simulink model "simple_dsp_module"  (R2018a)
settings: Solver=VariableStepAuto  StartTime=0.0  StopTime=100e-6  RelTol=1e-3
values from neighbouring files (symbols this model uses):
  BASELINE = 0    [dsp_blr.mat]
libraries: xbsIndex_r4 x84, xrbsSSR_Library x15, simulink x3, dspsigattribs x1, hdlsllib x1
(part 2 of 2)

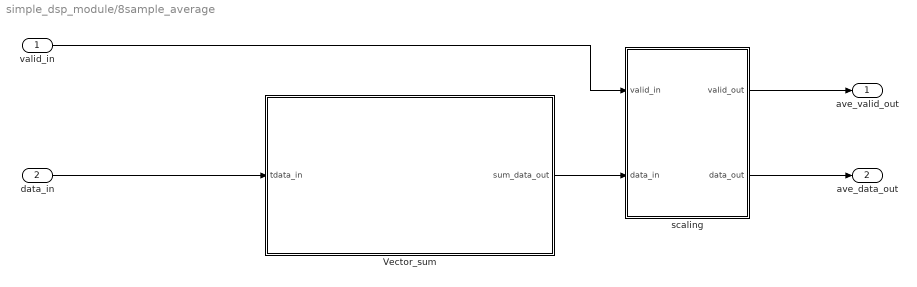
== system simple_dsp_module/8sample_average  ==
  valid_in : Inport
  data_in : Inport  Port=2
  Vector_sum : Subsystem
  scaling : Subsystem
  ave_valid_out : Outport
  ave_data_out : Outport  Port=2
  wires:
  valid_in/1 -> scaling/1(valid_in)
  Vector_sum/1(sum_data_out) -> scaling/2(data_in)
  scaling/2(data_out) -> ave_data_out/1
  data_in/1 -> Vector_sum/1(tdata_in)
  scaling/1(valid_out) -> ave_valid_out/1

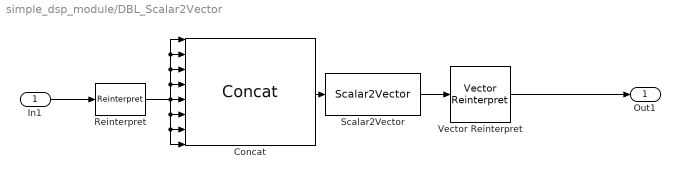
== system simple_dsp_module/DBL_Scalar2Vector ==
  In1 : Inport
  Concat : xbsIndex_r4/Concat  num_inputs=8  dbl_ovrd=off  block_type=concat
  Reinterpret : xbsIndex_r4/Reinterpret  force_arith_type=on  arith_type=Unsigned  force_bin_pt=on  bin_pt=0  block_type=reinterpret
  Scalar2Vector : xrbsSSR_Library/Scalar2Vector  Width=16  sg_ssr=8  sg_ssr_prev=8  sg_ssr_name=vect_Scalar2Vector  block_type=scalar2vector_ssr
      settings: SourceProductName=Xilinx SSR Blockset
  Vector Reinterpret : xrbsSSR_Library/Vector Reinterpret  sg_ssr=8  sg_ssr_prev=8  force_arith_type=on  arith_type="Signed  (2's comp)"  force_bin_pt=on  bin_pt=4  block_type=reinterpret_ssr
      settings: SourceProductName=Xilinx SSR Blockset  infoedit="The Vector Reinterpret block Changes vector input signal type without altering the binary representation. You can change the signal between signed and unsigned, and relocate the binary point.<br><br>Hardware notes: In hardware this block costs nothing.<br><br>Example:  Suppose the input is 6 bits wide, signed, with 2 fractional bits, and the output is forced to unsigned with 0 fractional bits.  Then an input of -2.0 (1110.00 in binary 2's complement) becomes an output of 56 (111000 in binary)."
  Out1 : Outport
  wires:
  In1/1 -> Reinterpret/1
  Vector Reinterpret/1 -> Out1/1
  Reinterpret/1 -> Concat/1, Concat/2, Concat/3, Concat/4, Concat/8, Concat/7, Concat/6, Concat/5
  Concat/1 -> Scalar2Vector/1
  Scalar2Vector/1 -> Vector Reinterpret/1

== system simple_dsp_module/DSP_Vector2Scalar ==
  In1 : Inport
  Vector2Scalar : xrbsSSR_Library/Vector2Scalar  sg_ssr=8  sg_ssr_prev=8  sg_ssr_name=vect_Vector2Scalar  block_type=vector2scalar_ssr
      settings: SourceProductName=Xilinx SSR Blockset
  Vector_reinterpret2unsigned : xrbsSSR_Library/Vector Reinterpret  sg_ssr=8  sg_ssr_prev=8  force_arith_type=on  arith_type=Unsigned  force_bin_pt=on  bin_pt=0  block_type=reinterpret_ssr
      settings: SourceProductName=Xilinx SSR Blockset  infoedit="The Vector Reinterpret block Changes vector input signal type without altering the binary representation. You can change the signal between signed and unsigned, and relocate the binary point.<br><br>Hardware notes: In hardware this block costs nothing.<br><br>Example:  Suppose the input is 6 bits wide, signed, with 2 fractional bits, and the output is forced to unsigned with 0 fractional bits.  Then an input of -2.0 (1110.00 in binary 2's complement) becomes an output of 56 (111000 in binary)."
  Out1 : Outport
  wires:
  Vector_reinterpret2unsigned/1 -> Vector2Scalar/1
  In1/1 -> Vector_reinterpret2unsigned/1
  Vector2Scalar/1 -> Out1/1

== system simple_dsp_module/HGAIN_Vector2Scalar ==
  In1 : Inport
  Vector2Scalar : xrbsSSR_Library/Vector2Scalar  sg_ssr=8  sg_ssr_prev=8  sg_ssr_name=vect_Vector2Scalar  block_type=vector2scalar_ssr
      settings: SourceProductName=Xilinx SSR Blockset
  Vector_reinterpret2unsigned : xrbsSSR_Library/Vector Reinterpret  sg_ssr=8  sg_ssr_prev=8  force_arith_type=on  arith_type=Unsigned  force_bin_pt=on  bin_pt=0  block_type=reinterpret_ssr
      settings: SourceProductName=Xilinx SSR Blockset  infoedit="The Vector Reinterpret block Changes vector input signal type without altering the binary representation. You can change the signal between signed and unsigned, and relocate the binary point.<br><br>Hardware notes: In hardware this block costs nothing.<br><br>Example:  Suppose the input is 6 bits wide, signed, with 2 fractional bits, and the output is forced to unsigned with 0 fractional bits.  Then an input of -2.0 (1110.00 in binary 2's complement) becomes an output of 56 (111000 in binary)."
  Out1 : Outport
  wires:
  Vector_reinterpret2unsigned/1 -> Vector2Scalar/1
  In1/1 -> Vector_reinterpret2unsigned/1
  Vector2Scalar/1 -> Out1/1

== system simple_dsp_module/Vector2Bus ==
  In1 : Inport
  Bit Concat : hdlsllib/Logic and Bit Operations/Bit Concat  numInputs=8
      settings: SourceProductName=HDL Coder  SourceProductBaseCode=HD
  Demux : Demux  Outputs=8
  Out1 : Outport
  wires:
  Demux/1 -> Bit Concat/8
  Demux/8 -> Bit Concat/1
  Demux/3 -> Bit Concat/6
  Bit Concat/1 -> Out1/1
  Demux/7 -> Bit Concat/2
  Demux/4 -> Bit Concat/5
  Demux/2 -> Bit Concat/7
  Demux/6 -> Bit Concat/3
  Demux/5 -> Bit Concat/4
  In1/1 -> Demux/1

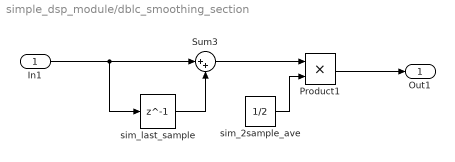
== system simple_dsp_module/dblc_smoothing_section ==
  In1 : Inport
  Product1 : Product
  Sum3 : Sum  Inputs=|++
  sim_2sample_ave : Constant  Value=1/2  VectorParams1D=off  OutDataTypeStr=Inherit: Inherit via back propagation  SampleTime=1/125e6
  sim_last_sample : Delay  DelayLength=1  InitialCondition=0
  Out1 : Outport
  wires:
  In1/1 -> sim_last_sample/1, Sum3/1
  sim_2sample_ave/1 -> Product1/2
  sim_last_sample/1 -> Sum3/2
  Sum3/1 -> Product1/1
  Product1/1 -> Out1/1

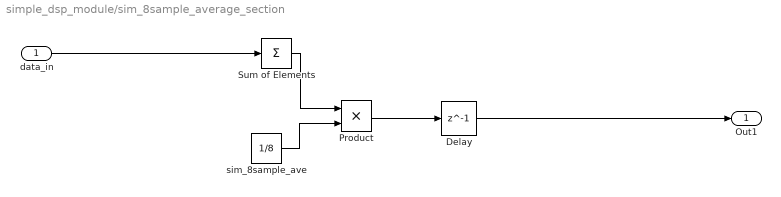
== system simple_dsp_module/sim_8sample_average_section ==
  data_in : Inport
  Delay : Delay  DelayLength=1  InitialCondition=0
  Product : Product
  Sum of Elements : Sum  Inputs=+
  sim_8sample_ave : Constant  Value=1/8  VectorParams1D=off  OutDataTypeStr=Inherit: Inherit via back propagation  SampleTime=1/125e6
  Out1 : Outport
  wires:
  data_in/1 -> Sum of Elements/1
  Sum of Elements/1 -> Product/1
  sim_8sample_ave/1 -> Product/2
  Product/1 -> Delay/1
  Delay/1 -> Out1/1

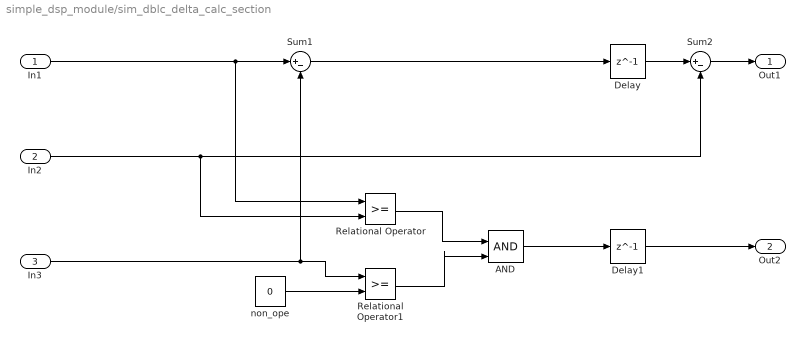
== system simple_dsp_module/sim_dblc_delta_calc_section ==
  In1 : Inport
  In2 : Inport  Port=2
  In3 : Inport  Port=3
  AND : Logic  IconShape=distinctive  AllPortsSameDT=off  OutDataTypeStr=boolean
  Delay : Delay  DelayLength=1  InitialCondition=0  InputProcessing=Columns as channels (frame based)
  Delay1 : Delay  DelayLength=1  InitialCondition=0  InputProcessing=Columns as channels (frame based)
  Relational Operator : RelationalOperator  OutDataTypeStr=boolean  RndMeth=Simplest
  Relational Operator1 : RelationalOperator  OutDataTypeStr=boolean  RndMeth=Simplest
  Sum1 : Sum  Inputs=|+-
  Sum2 : Sum  Inputs=|+-
  non_ope : Constant  Value=0  VectorParams1D=off  OutDataTypeStr=Inherit: Inherit via back propagation  SampleTime=1/125e6
  Out1 : Outport
  Out2 : Outport  Port=2
  wires:
  Sum2/1 -> Out1/1
  In1/1 -> Sum1/1, Relational Operator/1
  In2/1 -> Relational Operator/2, Sum2/2
  Relational Operator/1 -> AND/1
  AND/1 -> Delay1/1
  non_ope/1 -> Relational Operator1/2
  In3/1 -> Sum1/2, Relational Operator1/1
  Relational Operator1/1 -> AND/2
  Sum1/1 -> Delay/1
  Delay/1 -> Sum2/1
  Delay1/1 -> Out2/1

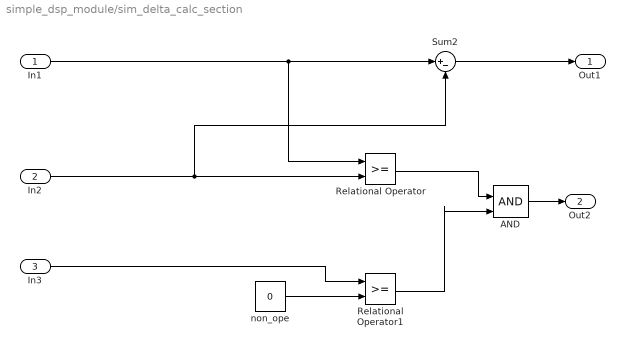
== system simple_dsp_module/sim_delta_calc_section ==
  In1 : Inport
  In2 : Inport  Port=2
  In3 : Inport  Port=3
  AND : Logic  IconShape=distinctive  AllPortsSameDT=off  OutDataTypeStr=boolean
  Relational Operator : RelationalOperator  OutDataTypeStr=boolean  RndMeth=Simplest
  Relational Operator1 : RelationalOperator  OutDataTypeStr=boolean  RndMeth=Simplest
  Sum2 : Sum  Inputs=|+-
  non_ope : Constant  Value=0  VectorParams1D=off  OutDataTypeStr=Inherit: Inherit via back propagation  SampleTime=1/125e6
  Out1 : Outport
  Out2 : Outport  Port=2
  wires:
  In1/1 -> Relational Operator/1, Sum2/1
  In2/1 -> Relational Operator/2, Sum2/2
  Relational Operator/1 -> AND/1
  AND/1 -> Out2/1
  non_ope/1 -> Relational Operator1/2
  In3/1 -> Relational Operator1/1
  Relational Operator1/1 -> AND/2
  Sum2/1 -> Out1/1

== system simple_dsp_module/smoothing_section ==
  In1 : Inport
  Product1 : Product
  Sum3 : Sum  Inputs=|++
  sim_2sample_ave : Constant  Value=1/2  VectorParams1D=off  OutDataTypeStr=Inherit: Inherit via back propagation  SampleTime=1/125e6
  sim_last_sample : Delay  DelayLength=1  InitialCondition=0
  Out1 : Outport
  wires:
  In1/1 -> sim_last_sample/1, Sum3/1
  sim_2sample_ave/1 -> Product1/2
  sim_last_sample/1 -> Sum3/2
  Sum3/1 -> Product1/1
  Product1/1 -> Out1/1

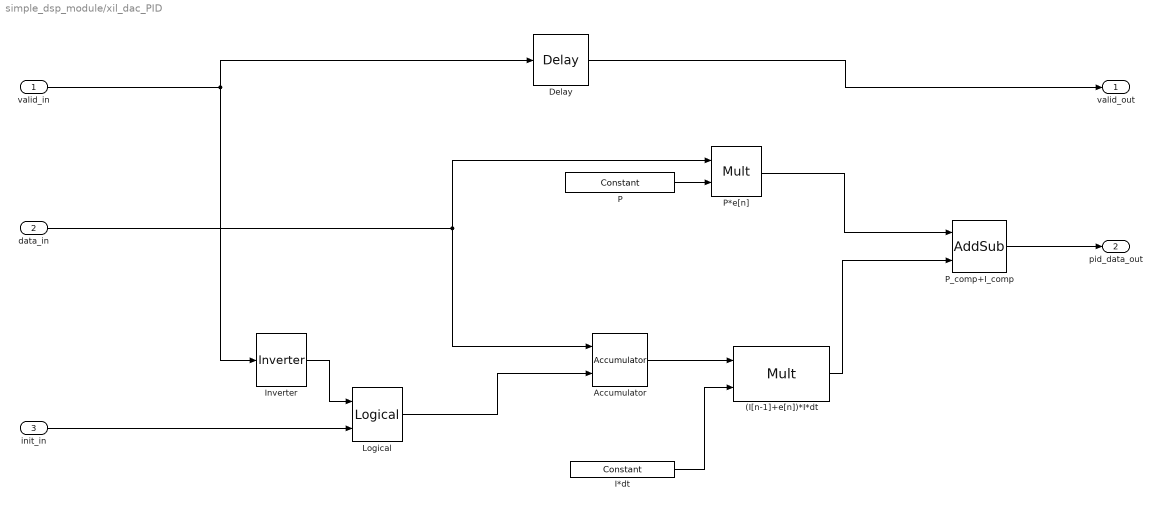
== system simple_dsp_module/xil_dac_PID ==
  valid_in : Inport
  data_in : Inport  Port=2
  init_in : Inport  Port=3
  (I[n-1]+e[n])*I*dt : xbsIndex_r4/Mult  precision=Full  arith_type="Signed  (2's comp)"  n_bits=36  bin_pt=22  quantization=Truncate  overflow=Wrap  en=off  latency=3  use_behavioral_HDL=off  opt=Speed  use_embedded=on  optimum_pipeline=off  pipeline=on  dbl_ovrd=off  use_rpm=on  placement_style=Triangular  block_type=mult
  Accumulator : xbsIndex_r4/Accumulator  operation=Add  n_bits=32  overflow=Wrap  scale=1  rst=on  hasbypass=on  infoeditControl=reset for floating point data type must be asserted for a minimum of 2 cycles  en=off  latency=1  msb_inp=100  msb=100  lsb=-100  use_behavioral_HDL=on  implementation=Fabric  dbl_ovrd=off  block_type=accum
  Delay : xbsIndex_r4/Delay  rst=off  infoeditControl=Selection of Reset will increase slice count due to use of real FFs and instead of SRLs  en=off  latency=4  reg_retiming=off  dbl_ovrd=off  block_type=delay
  I*dt : xbsIndex_r4/Constant  const=1826449.3603705*8e-9  gui_display_data_type=Fixed-point  arith_type=Signed (2's comp)  n_bits=16  bin_pt=16  preci_type=Single  exp_width=8  frac_width=24  explicit_period=off  period=1  equ=P=C  opselect=C  inp2=PCIN>>17  opr=+  inp1=P  carry=CIN  dbl_ovrd=off  block_type=constant
  Inverter : xbsIndex_r4/Inverter  en=off  latency=0  dbl_ovrd=off  block_type=inv
  Logical : xbsIndex_r4/Logical  logical_function=OR  inputs=2  en=off  latency=0  precision=Full  arith_type=Unsigned  n_bits=16  bin_pt=0  align_bp=on  dbl_ovrd=off  block_type=logical
  P : xbsIndex_r4/Constant  const=0.00730579744148201  gui_display_data_type=Fixed-point  arith_type=Signed (2's comp)  n_bits=16  bin_pt=16  preci_type=Single  exp_width=8  frac_width=24  explicit_period=off  period=1  equ=P=C  opselect=C  inp2=PCIN>>17  opr=+  inp1=P  carry=CIN  dbl_ovrd=off  block_type=constant
  P*e[n] : xbsIndex_r4/Mult  precision=Full  arith_type="Signed  (2's comp)"  n_bits=16  bin_pt=14  quantization=Truncate  overflow=Wrap  en=off  latency=3  use_behavioral_HDL=off  opt=Speed  use_embedded=on  optimum_pipeline=off  pipeline=on  dbl_ovrd=off  use_rpm=on  placement_style=Triangular  block_type=mult
  P_comp+I_comp : xbsIndex_r4/AddSub  mode=Addition  use_carryin=off  use_carryout=off  en=off  latency=0  precision=Full  arith_type=Unsigned  n_bits=16  bin_pt=4  quantization=Truncate  overflow=Wrap  use_behavioral_HDL=off  hw_selection=Fabric  pipelined=off  dbl_ovrd=off  block_type=addsub
  valid_out : Outport
  pid_data_out : Outport  Port=2
  wires:
  P_comp+I_comp/1 -> pid_data_out/1
  data_in/1 -> P*e[n]/1, Accumulator/1
  I*dt/1 -> (I[n-1]+e[n])*I*dt/2
  (I[n-1]+e[n])*I*dt/1 -> P_comp+I_comp/2
  P/1 -> P*e[n]/2
  P*e[n]/1 -> P_comp+I_comp/1
  valid_in/1 -> Delay/1, Inverter/1
  Accumulator/1 -> (I[n-1]+e[n])*I*dt/1
  Logical/1 -> Accumulator/2
  init_in/1 -> Logical/2
  Inverter/1 -> Logical/1
  Delay/1 -> valid_out/1

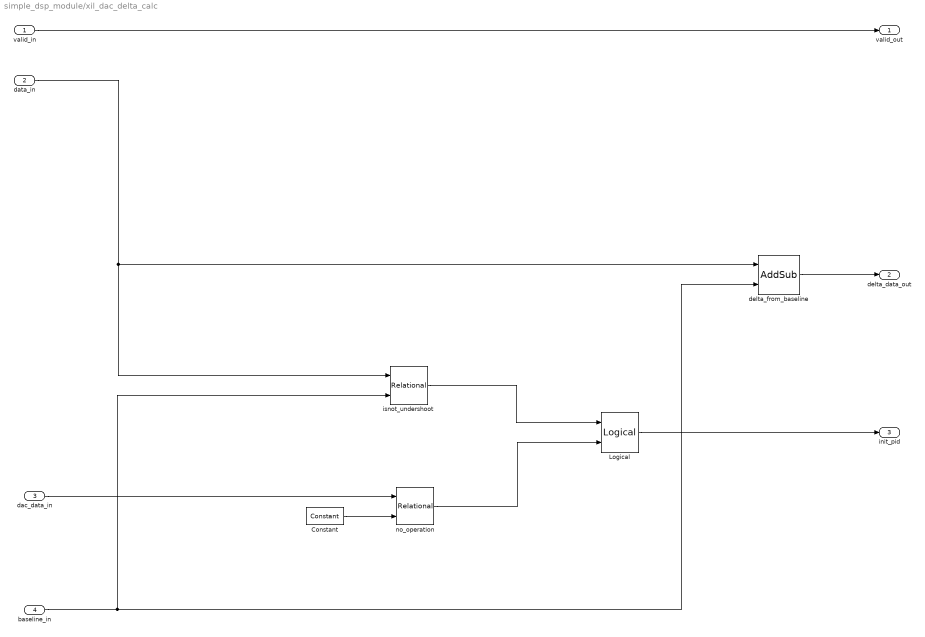
== system simple_dsp_module/xil_dac_delta_calc ==
  valid_in : Inport
  data_in : Inport  Port=2
  dac_data_in : Inport  Port=3
  baseline_in : Inport  Port=4
  Constant : xbsIndex_r4/Constant  const=0  gui_display_data_type=Fixed-point  arith_type=Signed (2's comp)  n_bits=16  bin_pt=4  preci_type=Single  exp_width=8  frac_width=24  explicit_period=off  period=1  equ=P=C  opselect=C  inp2=PCIN>>17  opr=+  inp1=P  carry=CIN  dbl_ovrd=off  block_type=constant
  Logical : xbsIndex_r4/Logical  logical_function=AND  inputs=2  en=off  latency=0  precision=User Defined  arith_type=Boolean  n_bits=1  bin_pt=0  align_bp=on  dbl_ovrd=off  block_type=logical
  delta_from_baseline : xbsIndex_r4/AddSub  mode=Subtraction  use_carryin=off  use_carryout=off  en=off  latency=0  precision=Full  arith_type=Unsigned  n_bits=16  bin_pt=14  quantization=Truncate  overflow=Wrap  use_behavioral_HDL=off  hw_selection=Fabric  pipelined=off  dbl_ovrd=off  block_type=addsub
  isnot_undershoot : xbsIndex_r4/Relational  mode=a>b  op_type=Bool  en=off  latency=0  dbl_ovrd=off  block_type=relational
  no_operation : xbsIndex_r4/Relational  mode=a>b  op_type=Bool  en=off  latency=0  dbl_ovrd=off  block_type=relational
  valid_out : Outport
  delta_data_out : Outport  Port=2
  init_pid : Outport  Port=3
  wires:
  delta_from_baseline/1 -> delta_data_out/1
  valid_in/1 -> valid_out/1
  isnot_undershoot/1 -> Logical/1
  Constant/1 -> no_operation/2
  dac_data_in/1 -> no_operation/1
  no_operation/1 -> Logical/2
  Logical/1 -> init_pid/1
  baseline_in/1 -> isnot_undershoot/2, delta_from_baseline/2
  data_in/1 -> delta_from_baseline/1, isnot_undershoot/1

== system simple_dsp_module/xil_dac_smoothing ==
  data_in : Inport
  2sample_ave : xbsIndex_r4/Shift  shift_dir=Right  shift_bits=1  en=off  latency=0  precision=Full  arith_type="Signed  (2's comp)"  n_bits=16  bin_pt=14  quantization=Truncate  overflow=Wrap  dbl_ovrd=off  block_type=shift
  2sample_sum : xbsIndex_r4/AddSub  mode=Addition  use_carryin=off  use_carryout=off  en=off  latency=0  precision=Full  arith_type=Unsigned  n_bits=16  bin_pt=14  quantization=Truncate  overflow=Wrap  use_behavioral_HDL=off  hw_selection=Fabric  pipelined=off  dbl_ovrd=off  block_type=addsub
  last_sample : xbsIndex_r4/Delay  rst=off  infoeditControl=Selection of Reset will increase slice count due to use of real FFs and instead of SRLs  en=off  latency=1  reg_retiming=off  dbl_ovrd=off  block_type=delay
  data_out : Outport
  wires:
  last_sample/1 -> 2sample_sum/2
  data_in/1 -> last_sample/1, 2sample_sum/1
  2sample_sum/1 -> 2sample_ave/1
  2sample_ave/1 -> data_out/1

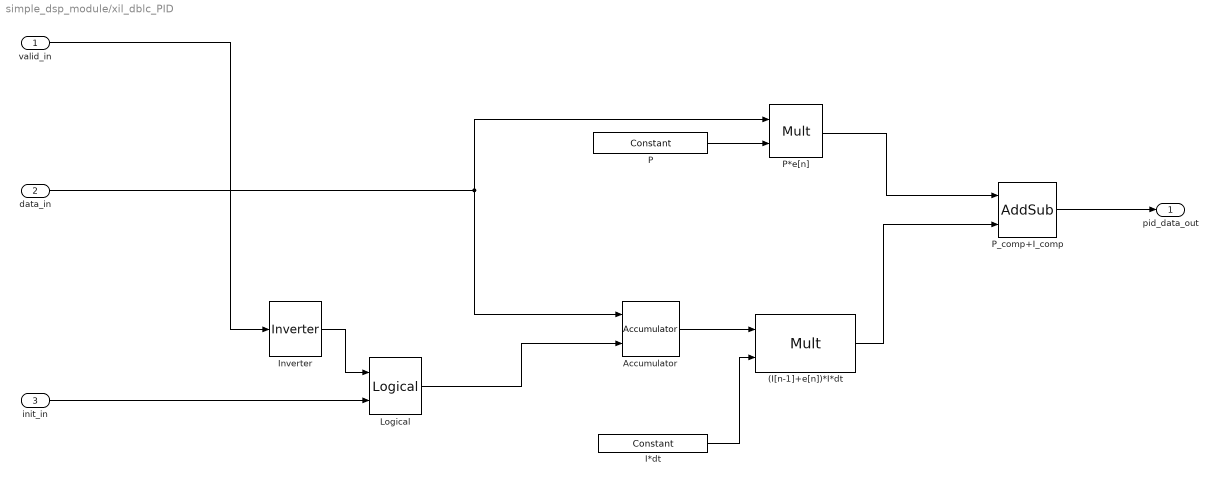
== system simple_dsp_module/xil_dblc_PID ==
  valid_in : Inport
  data_in : Inport  Port=2
  init_in : Inport  Port=3
  (I[n-1]+e[n])*I*dt : xbsIndex_r4/Mult  precision=Full  arith_type="Signed  (2's comp)"  n_bits=36  bin_pt=22  quantization=Truncate  overflow=Wrap  en=off  latency=3  use_behavioral_HDL=off  opt=Speed  use_embedded=on  optimum_pipeline=off  pipeline=on  dbl_ovrd=off  use_rpm=on  placement_style=Triangular  block_type=mult
  Accumulator : xbsIndex_r4/Accumulator  operation=Add  n_bits=32  overflow=Wrap  scale=1  rst=on  hasbypass=on  infoeditControl=reset for floating point data type must be asserted for a minimum of 2 cycles  en=off  latency=1  msb_inp=100  msb=100  lsb=-100  use_behavioral_HDL=on  implementation=Fabric  dbl_ovrd=off  block_type=accum
  I*dt : xbsIndex_r4/Constant  const=1826449.3603705*8e-9  gui_display_data_type=Fixed-point  arith_type=Signed (2's comp)  n_bits=16  bin_pt=16  preci_type=Single  exp_width=8  frac_width=24  explicit_period=off  period=1  equ=P=C  opselect=C  inp2=PCIN>>17  opr=+  inp1=P  carry=CIN  dbl_ovrd=off  block_type=constant
  Inverter : xbsIndex_r4/Inverter  en=off  latency=0  dbl_ovrd=off  block_type=inv
  Logical : xbsIndex_r4/Logical  logical_function=OR  inputs=2  en=off  latency=0  precision=Full  arith_type=Unsigned  n_bits=16  bin_pt=0  align_bp=on  dbl_ovrd=off  block_type=logical
  P : xbsIndex_r4/Constant  const=0.00730579744148201  gui_display_data_type=Fixed-point  arith_type=Signed (2's comp)  n_bits=16  bin_pt=16  preci_type=Single  exp_width=8  frac_width=24  explicit_period=off  period=1  equ=P=C  opselect=C  inp2=PCIN>>17  opr=+  inp1=P  carry=CIN  dbl_ovrd=off  block_type=constant
  P*e[n] : xbsIndex_r4/Mult  precision=Full  arith_type="Signed  (2's comp)"  n_bits=16  bin_pt=14  quantization=Truncate  overflow=Wrap  en=off  latency=3  use_behavioral_HDL=off  opt=Speed  use_embedded=on  optimum_pipeline=off  pipeline=on  dbl_ovrd=off  use_rpm=on  placement_style=Triangular  block_type=mult
  P_comp+I_comp : xbsIndex_r4/AddSub  mode=Addition  use_carryin=off  use_carryout=off  en=off  latency=0  precision=Full  arith_type=Unsigned  n_bits=16  bin_pt=4  quantization=Truncate  overflow=Wrap  use_behavioral_HDL=off  hw_selection=Fabric  pipelined=off  dbl_ovrd=off  block_type=addsub
  pid_data_out : Outport
  wires:
  P_comp+I_comp/1 -> pid_data_out/1
  data_in/1 -> P*e[n]/1, Accumulator/1
  I*dt/1 -> (I[n-1]+e[n])*I*dt/2
  (I[n-1]+e[n])*I*dt/1 -> P_comp+I_comp/2
  P/1 -> P*e[n]/2
  P*e[n]/1 -> P_comp+I_comp/1
  valid_in/1 -> Inverter/1
  Accumulator/1 -> (I[n-1]+e[n])*I*dt/1
  Logical/1 -> Accumulator/2
  init_in/1 -> Logical/2
  Inverter/1 -> Logical/1

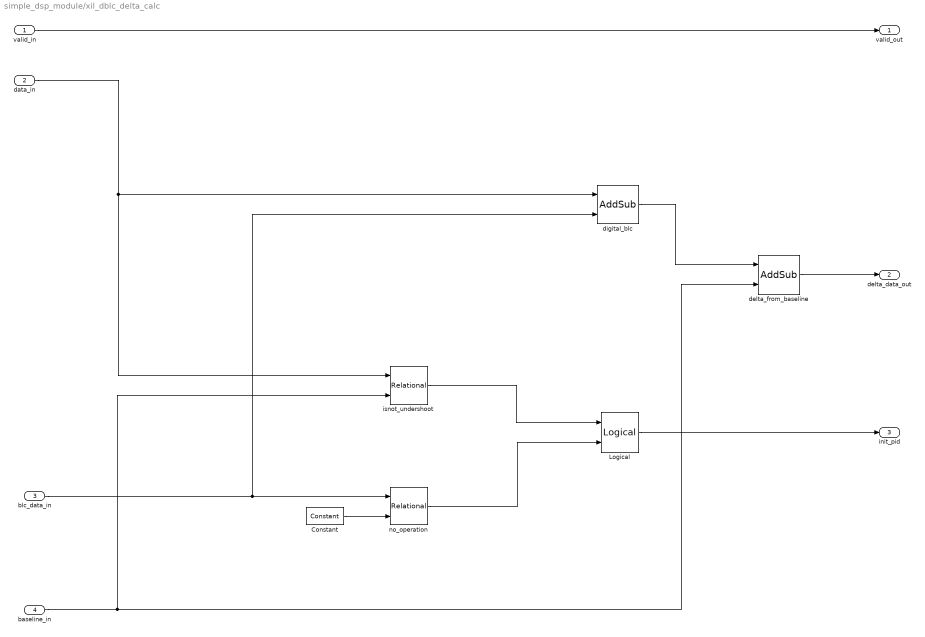
== system simple_dsp_module/xil_dblc_delta_calc ==
  valid_in : Inport
  data_in : Inport  Port=2
  blc_data_in : Inport  Port=3
  baseline_in : Inport  Port=4
  Constant : xbsIndex_r4/Constant  const=0  gui_display_data_type=Fixed-point  arith_type=Signed (2's comp)  n_bits=16  bin_pt=4  preci_type=Single  exp_width=8  frac_width=24  explicit_period=off  period=1  equ=P=C  opselect=C  inp2=PCIN>>17  opr=+  inp1=P  carry=CIN  dbl_ovrd=off  block_type=constant
  Logical : xbsIndex_r4/Logical  logical_function=AND  inputs=2  en=off  latency=1  precision=User Defined  arith_type=Boolean  n_bits=1  bin_pt=0  align_bp=on  dbl_ovrd=off  block_type=logical
  delta_from_baseline : xbsIndex_r4/AddSub  mode=Subtraction  use_carryin=off  use_carryout=off  en=off  latency=0  precision=Full  arith_type=Unsigned  n_bits=16  bin_pt=14  quantization=Truncate  overflow=Wrap  use_behavioral_HDL=off  hw_selection=Fabric  pipelined=off  dbl_ovrd=off  block_type=addsub
  digital_blc : xbsIndex_r4/AddSub  mode=Subtraction  use_carryin=off  use_carryout=off  en=off  latency=1  precision=Full  arith_type=Unsigned  n_bits=16  bin_pt=14  quantization=Truncate  overflow=Wrap  use_behavioral_HDL=off  hw_selection=Fabric  pipelined=off  dbl_ovrd=off  block_type=addsub
  isnot_undershoot : xbsIndex_r4/Relational  mode=a>b  op_type=Bool  en=off  latency=0  dbl_ovrd=off  block_type=relational
  no_operation : xbsIndex_r4/Relational  mode=a>b  op_type=Bool  en=off  latency=0  dbl_ovrd=off  block_type=relational
  valid_out : Outport
  delta_data_out : Outport  Port=2
  init_pid : Outport  Port=3
  wires:
  data_in/1 -> isnot_undershoot/1, digital_blc/1
  delta_from_baseline/1 -> delta_data_out/1
  valid_in/1 -> valid_out/1
  isnot_undershoot/1 -> Logical/1
  Constant/1 -> no_operation/2
  blc_data_in/1 -> digital_blc/2, no_operation/1
  no_operation/1 -> Logical/2
  Logical/1 -> init_pid/1
  baseline_in/1 -> isnot_undershoot/2, delta_from_baseline/2
  digital_blc/1 -> delta_from_baseline/1

== system simple_dsp_module/xil_dblc_smoothing ==
  data_in : Inport
  2sample_ave : xbsIndex_r4/Shift  shift_dir=Right  shift_bits=1  en=off  latency=0  precision=Full  arith_type="Signed  (2's comp)"  n_bits=16  bin_pt=14  quantization=Truncate  overflow=Wrap  dbl_ovrd=off  block_type=shift
  2sample_sum : xbsIndex_r4/AddSub  mode=Addition  use_carryin=off  use_carryout=off  en=off  latency=0  precision=Full  arith_type=Unsigned  n_bits=16  bin_pt=14  quantization=Truncate  overflow=Wrap  use_behavioral_HDL=off  hw_selection=Fabric  pipelined=off  dbl_ovrd=off  block_type=addsub
  last_sample : xbsIndex_r4/Delay  rst=off  infoeditControl=Selection of Reset will increase slice count due to use of real FFs and instead of SRLs  en=off  latency=1  reg_retiming=off  dbl_ovrd=off  block_type=delay
  data_out : Outport
  wires:
  last_sample/1 -> 2sample_sum/2
  data_in/1 -> last_sample/1, 2sample_sum/1
  2sample_sum/1 -> 2sample_ave/1
  2sample_ave/1 -> data_out/1

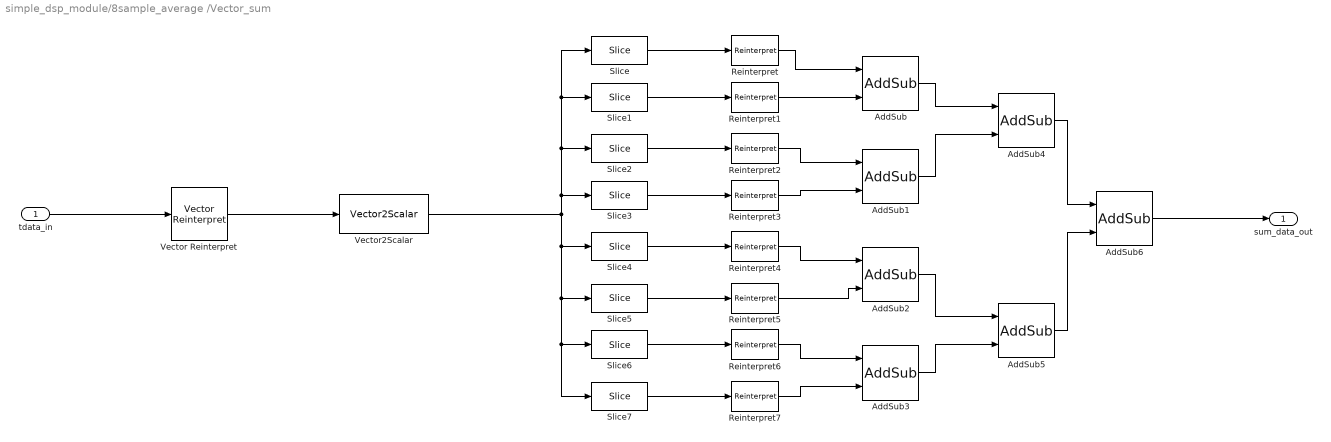
== system simple_dsp_module/8sample_average /Vector_sum ==
  tdata_in : Inport
  AddSub{,1..3} (4 alike) : xbsIndex_r4/AddSub  mode=Addition  use_carryin=off  use_carryout=off  en=off  latency=0  precision=User Defined  arith_type="Signed  (2's comp)"  n_bits=17  bin_pt=4  quantization=Truncate  overflow=Wrap  use_behavioral_HDL=off  hw_selection=Fabric  pipelined=off  dbl_ovrd=off  block_type=addsub
  AddSub4 : xbsIndex_r4/AddSub  mode=Addition  use_carryin=off  use_carryout=off  en=off  latency=0  precision=Full  arith_type="Signed  (2's comp)"  n_bits=18  bin_pt=4  quantization=Truncate  overflow=Wrap  use_behavioral_HDL=off  hw_selection=Fabric  pipelined=off  dbl_ovrd=off  block_type=addsub
  AddSub5 : xbsIndex_r4/AddSub  mode=Addition  use_carryin=off  use_carryout=off  en=off  latency=0  precision=Full  arith_type="Signed  (2's comp)"  n_bits=18  bin_pt=4  quantization=Truncate  overflow=Wrap  use_behavioral_HDL=off  hw_selection=Fabric  pipelined=off  dbl_ovrd=off  block_type=addsub
  AddSub6 : xbsIndex_r4/AddSub  mode=Addition  use_carryin=off  use_carryout=off  en=off  latency=0  precision=User Defined  arith_type="Signed  (2's comp)"  n_bits=19  bin_pt=4  quantization=Truncate  overflow=Wrap  use_behavioral_HDL=off  hw_selection=Fabric  pipelined=off  dbl_ovrd=off  block_type=addsub
  Reinterpret{,1..7} (8 alike) : xbsIndex_r4/Reinterpret  force_arith_type=on  arith_type="Signed  (2's comp)"  force_bin_pt=on  bin_pt=4  block_type=reinterpret
  Slice : xbsIndex_r4/Slice  nbits=16  boolean_output=off  mode=Two Bit Locations  bit1=15  base1=LSB of Input  bit0=0  base0=LSB of Input  dbl_ovrd=off  block_type=slice
  Slice1 : xbsIndex_r4/Slice  nbits=16  boolean_output=off  mode=Two Bit Locations  bit1=31  base1=LSB of Input  bit0=16  base0=LSB of Input  dbl_ovrd=off  block_type=slice
  Slice2 : xbsIndex_r4/Slice  nbits=16  boolean_output=off  mode=Two Bit Locations  bit1=47  base1=LSB of Input  bit0=32  base0=LSB of Input  dbl_ovrd=off  block_type=slice
  Slice3 : xbsIndex_r4/Slice  nbits=16  boolean_output=off  mode=Two Bit Locations  bit1=63  base1=LSB of Input  bit0=48  base0=LSB of Input  dbl_ovrd=off  block_type=slice
  Slice4 : xbsIndex_r4/Slice  nbits=16  boolean_output=off  mode=Two Bit Locations  bit1=79  base1=LSB of Input  bit0=64  base0=LSB of Input  dbl_ovrd=off  block_type=slice
  Slice5 : xbsIndex_r4/Slice  nbits=16  boolean_output=off  mode=Two Bit Locations  bit1=95  base1=LSB of Input  bit0=80  base0=LSB of Input  dbl_ovrd=off  block_type=slice
  Slice6 : xbsIndex_r4/Slice  nbits=16  boolean_output=off  mode=Two Bit Locations  bit1=111  base1=LSB of Input  bit0=96  base0=LSB of Input  dbl_ovrd=off  block_type=slice
  Slice7 : xbsIndex_r4/Slice  nbits=16  boolean_output=off  mode=Two Bit Locations  bit1=127  base1=LSB of Input  bit0=112  base0=LSB of Input  dbl_ovrd=off  block_type=slice
  Vector Reinterpret : xrbsSSR_Library/Vector Reinterpret  sg_ssr=8  sg_ssr_prev=8  force_arith_type=on  arith_type=Unsigned  force_bin_pt=on  bin_pt=0  block_type=reinterpret_ssr
      settings: SourceProductName=Xilinx SSR Blockset  infoedit="The Vector Reinterpret block Changes vector input signal type without altering the binary representation. You can change the signal between signed and unsigned, and relocate the binary point.<br><br>Hardware notes: In hardware this block costs nothing.<br><br>Example:  Suppose the input is 6 bits wide, signed, with 2 fractional bits, and the output is forced to unsigned with 0 fractional bits.  Then an input of -2.0 (1110.00 in binary 2's complement) becomes an output of 56 (111000 in binary)."
  Vector2Scalar : xrbsSSR_Library/Vector2Scalar  sg_ssr=8  sg_ssr_prev=8  sg_ssr_name=vect_Vector2Scalar  block_type=vector2scalar_ssr
      settings: SourceProductName=Xilinx SSR Blockset
  sum_data_out : Outport  OutDataTypeStr=fixdt(1,19,4)
  wires:
  AddSub4/1 -> AddSub6/1
  Vector2Scalar/1 -> Slice7/1, Slice6/1, Slice5/1, Slice4/1, Slice2/1, Slice/1, Slice1/1, Slice3/1
  AddSub1/1 -> AddSub4/2
  AddSub5/1 -> AddSub6/2
  AddSub/1 -> AddSub4/1
  AddSub3/1 -> AddSub5/2
  AddSub2/1 -> AddSub5/1
  AddSub6/1 -> sum_data_out/1
  Slice/1 -> Reinterpret/1
  Slice1/1 -> Reinterpret1/1
  Slice2/1 -> Reinterpret2/1
  Slice3/1 -> Reinterpret3/1
  Slice4/1 -> Reinterpret4/1
  Slice5/1 -> Reinterpret5/1
  Slice6/1 -> Reinterpret6/1
  Slice7/1 -> Reinterpret7/1
  Reinterpret/1 -> AddSub/1
  Reinterpret1/1 -> AddSub/2
  Reinterpret2/1 -> AddSub1/1
  Reinterpret3/1 -> AddSub1/2
  Reinterpret4/1 -> AddSub2/1
  Reinterpret5/1 -> AddSub2/2
  Reinterpret6/1 -> AddSub3/1
  Reinterpret7/1 -> AddSub3/2
  tdata_in/1 -> Vector Reinterpret/1
  Vector Reinterpret/1 -> Vector2Scalar/1

== system simple_dsp_module/8sample_average /scaling ==
  valid_in : Inport
  data_in : Inport  Port=2
  Shift : xbsIndex_r4/Shift  shift_dir=Right  shift_bits=3  en=off  latency=1  precision=Full  arith_type="Signed  (2's comp)"  n_bits=16  bin_pt=14  quantization=Truncate  overflow=Wrap  dbl_ovrd=off  block_type=shift
  tvalid_delay : xbsIndex_r4/Delay  rst=off  infoeditControl=Selection of Reset will increase slice count due to use of real FFs and instead of SRLs  en=off  latency=1  reg_retiming=off  dbl_ovrd=off  block_type=delay
  valid_out : Outport
  data_out : Outport  Port=2
  wires:
  valid_in/1 -> tvalid_delay/1
  tvalid_delay/1 -> valid_out/1
  data_in/1 -> Shift/1
  Shift/1 -> data_out/1
